simulink model "DA3sim"  (R2018a)
settings: Solver=VariableStepAuto  StartTime=0.0  StopTime=5  RelTol=1e-3
values from neighbouring files (symbols this model uses):
  c = 60    [DA3run.m]
  k_s = 586.39    [DA3run.m]
  k_t = 10*k_s    (= 5863.9)    [DA3run.m]
  m_s = 0.437    [DA3run.m]
  m_u = 0.117    [DA3run.m]
  t_step = 0.0001    [DA3run.m]
settings Model: Creator=Chris  LastModifiedBy=sa2saiye
settings DebuggingCC: LibraryContextMissingDiagnostic=warning
settings SFSimCC: SimUseLocalCustomCode=on
settings RTWCC: RTWUseLocalCustomCode=on

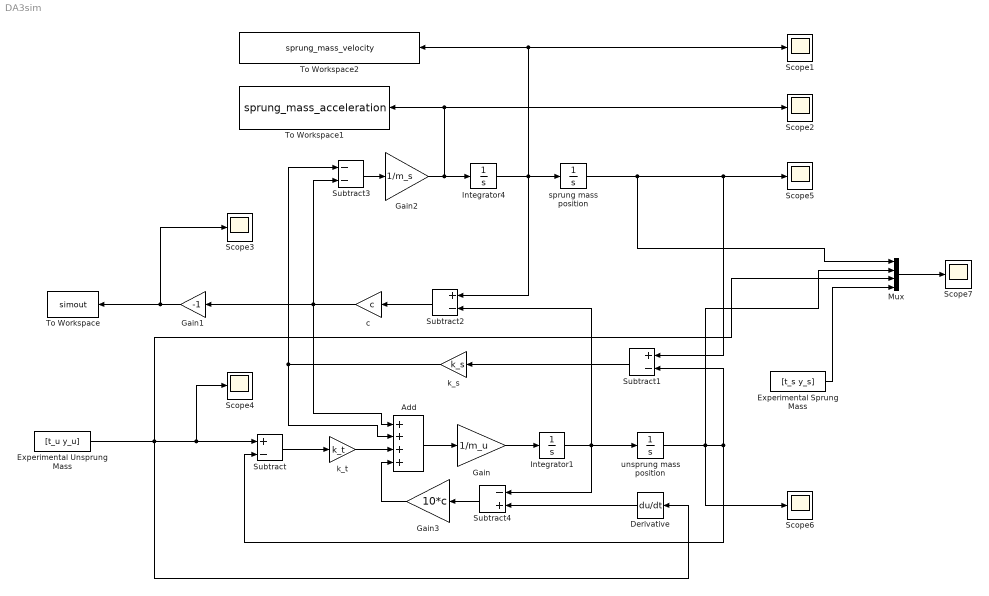
== system DA3sim ==
  Add : Sum  Inputs=++++
  Derivative : Derivative  CoefficientInTFapproximation=0
  Experimental Sprung Mass : FromWorkspace  VariableName=[t_s y_s]  SampleTime=t_step
  Experimental Unsprung Mass : FromWorkspace  VariableName=[t_u y_u]  SampleTime=t_step
  Gain : Gain  Gain=1/m_u
  Gain1 : Gain  Gain=-1
  Gain2 : Gain  Gain=1/m_s
  Gain3 : Gain  Gain=10*c
  Integrator1 : Integrator
  Integrator4 : Integrator
  Mux : Mux
  Scope{1..7} (7 alike) : Scope
  Subtract : Sum  Inputs=+-
  Subtract1 : Sum  Inputs=+-
  Subtract2 : Sum  Inputs=+-
  Subtract3 : Sum  Inputs=--
  Subtract4 : Sum  Inputs=-+
  To Workspace : ToWorkspace  VariableName=simout  SaveFormat=Timeseries  SampleTime=-1
  To Workspace1 : ToWorkspace  VariableName=sprung_mass_acceleration  SaveFormat=Timeseries  SampleTime=-1
  To Workspace2 : ToWorkspace  VariableName=sprung_mass_velocity  SaveFormat=Timeseries  SampleTime=-1
  c : Gain  Gain=c
  k_s : Gain  Gain=k_s
  k_t : Gain  Gain=k_t
  sprung mass position : Integrator
  unsprung mass position : Integrator
  wires:
  Add/1 -> Gain/1
  k_s/1 -> Add/2, Subtract3/1
  c/1 -> Add/1, Gain1/1, Subtract3/2
  Gain2/1 -> To Workspace1/1, Scope2/1, Integrator4/1
  Subtract/1 -> k_t/1
  Gain1/1 -> Scope3/1, To Workspace/1
  Integrator1/1 -> Subtract2/2, unsprung mass position/1, Subtract4/1
  Subtract1/1 -> k_s/1
  Subtract2/1 -> c/1
  sprung mass position/1 -> Mux/1, Scope5/1, Subtract1/1
  k_t/1 -> Add/3
  unsprung mass position/1 -> Subtract1/2, Subtract/2, Mux/2, Scope6/1
  Gain/1 -> Integrator1/1
  Integrator4/1 -> Subtract2/1, Scope1/1, To Workspace2/1, sprung mass position/1
  Subtract3/1 -> Gain2/1
  Mux/1 -> Scope7/1
  Subtract4/1 -> Gain3/1
  Gain3/1 -> Add/4
  Experimental Unsprung Mass/1 -> Scope4/1, Subtract/1, Derivative/1, Mux/3
  Derivative/1 -> Subtract4/2
  Experimental Sprung Mass/1 -> Mux/4
